simulink model "PIDcontroler"  (R2025b)
settings: Solver=VariableStepAuto  StartTime=0.0  StopTime=100  RelTol=1e-3
undefined symbols (not defined in the file): C_T_pitch, C_T_rol, C_T_yaw, Ix, Iy, Iz
libraries: slpidlib x3
settings Model: Creator=torcik  LastModifiedBy=torcik

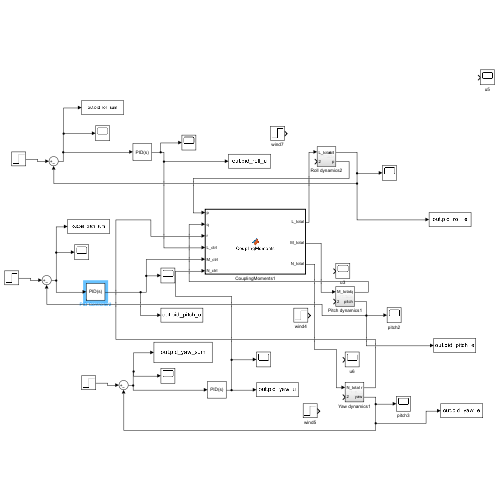
[thumbnail: Simulink's stored preview of the top-level diagram]
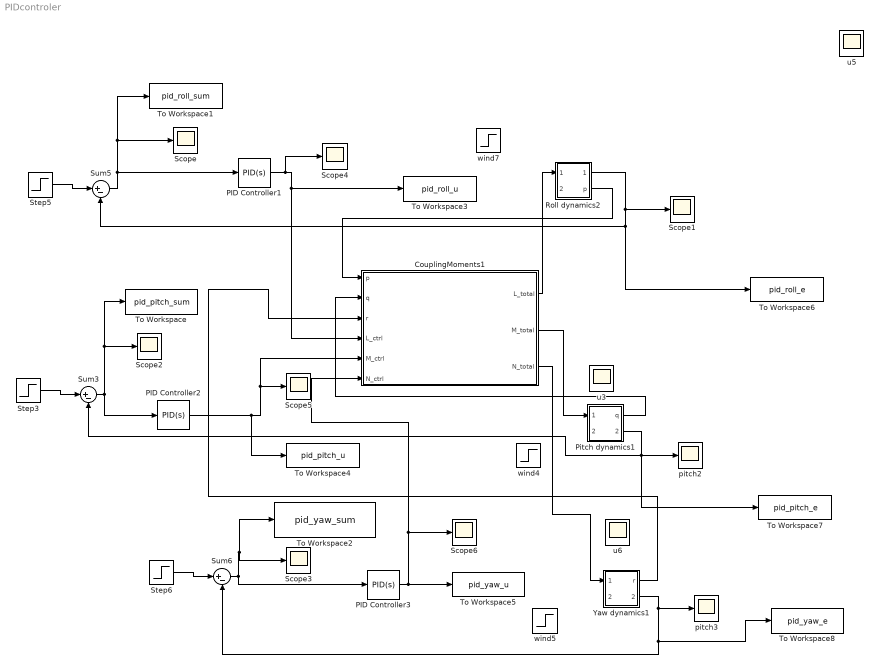
== system PIDcontroler ==
  CouplingMoments1 : MATLAB Function  TreatAsAtomicUnit=on
  PID Controller1 : slpidlib/PID Controller  Controller=PID  Form=Parallel  TimeDomain=Continuous-time  UseExternalTs=off  SampleTime=-1  IntegratorMethod=Forward Euler  FilterMethod=Forward Euler  ControllerParametersSource=internal  P=6.65  I=0.14  UseKiTs=off  D=15.6  UseExternalDerivativeSource=off  N=100  UseFilter=on  TunerSelectOption=Transfer Function Based (PID Tuner App)  InitialConditionSource=internal  InitialConditionForIntegrator=0  InitialConditionForFilter=0  DifferentiatorICPrevScaledInput=0  ExternalReset=none  TrackingMode=off  Kt=1  LimitOutput=off  SatLimitsSource=internal  UpperSaturationLimit=inf  LowerSaturationLimit=-inf  LinearizeAsGain=on  AntiWindupMode=none  Kb=1  LimitIntegrator=off  UpperIntegratorSaturationLimit=inf  LowerIntegratorSaturationLimit=-inf  POutMin=[]  POutMax=[]  IOutMin=[]  IOutMax=[]  DOutMin=[]  DOutMax=[]  NOutMin=[]  NOutMax=[]  SumOutMin=[]  SumOutMax=[]  SaturationOutMin=[]  SaturationOutMax=[]  PParamMin=[]  PParamMax=[]  IParamMin=[]  IParamMax=[]  DParamMin=[]  DParamMax=[]  NParamMin=[]  NParamMax=[]  KbParamMin=[]  KbParamMax=[]  KtParamMin=[]  KtParamMax=[]  KbOutMin=[]  KbOutMax=[]  KtOutMin=[]  KtOutMax=[]  IntegratorOutMin=[]  IntegratorOutMax=[]  FilterOutMin=[]  FilterOutMax=[]  SumI1OutMin=[]  SumI1OutMax=[]  SumI2OutMin=[]  SumI2OutMax=[]  SumI3OutMin=[]  SumI3OutMax=[]  SumI4OutMin=[]  SumI4OutMax=[]  SumDOutMin=[]  SumDOutMax=[]  DifferentiatorOutMin=[]  DifferentiatorOutMax=[]  FilterDiffOutCoefMin=[]  FilterDiffOutCoefMax=[]  ReciprocalOutMin=[]  ReciprocalOutMax=[]  SumDenOutMin=[]  SumDenOutMax=[]  SumNumOutMin=[]  SumNumOutMax=[]  DivideOutMin=[]  DivideOutMax=[]  UdiffTsProdOutMin=[]  UdiffTsProdOutMax=[]  NTsProdOutMin=[]  NTsProdOutMax=[]  UintegralTsProdOutMin=[]  UintegralTsProdOutMax=[]  UngainTsProdOutMin=[]  UngainTsProdOutMax=[]  ClampingZeroOutDataTypeStr=Inherit: Inherit via back propagation  ClampingZeroOutMin=[]  ClampingZeroOutMax=[]  FilterDenConstantOutDataTypeStr=Inherit: Inherit via back propagation  FilterDenConstantOutMin=[]  FilterDenConstantOutMax=[]  PCopyOutDataTypeStr=Inherit: Inherit via back propagation  PCopyOutMin=[]  PCopyOutMax=[]  NCopyOutDataTypeStr=Inherit: Inherit via back propagation  NCopyOutMin=[]  NCopyOutMax=[]  IntegratorContinuousStateAttributes=''  IntegratorStateMustResolveToSignalObject=off  IntegratorRTWStateStorageClass=Auto  FilterContinuousStateAttributes=''  FilterStateMustResolveToSignalObject=off  FilterRTWStateStorageClass=Auto  ParallelPVariant=InternalParameters  IdealPVariant=Disabled  IVariant=InternalParameters  DVariant=InternalParameters  IntegratorVariant=Continuous  SatVariant=Disabled  AWVariant=Passthrough  PCopyVariant=Disabled  TRVariant=Disabled  FdbkBlocksVariant=Forward  IdealPFdbkVariant=Disabled  SatFdbkVariant=Disabled  DerivativeFilterVariant=ContFilter  NVariant=InternalParameters  NCopyVariant=Disabled  FilterICVariant=InternalICsFilter  IntegratorICVariant=InternalICs  ExternalResetVariant=Disabled  TRSumVariant=Passthrough  SumFdbkVariant=Disabled  SumVariant=Sum_PID  TsampFilterVariant=InternalTs  TsampNgainVariant=Passthrough  TsampIntegralVariant=Disabled_SignalSpec  ExternalSaturationOutDataTypeStr=Inherit: Same as second input  DerivativeSourceVariant=ErrorSignal  PreIntVariant=InternalPreInt
  PID Controller2 : slpidlib/PID Controller  Controller=PID  Form=Parallel  TimeDomain=Continuous-time  UseExternalTs=off  SampleTime=-1  IntegratorMethod=Forward Euler  FilterMethod=Forward Euler  ControllerParametersSource=internal  P=9.74  I=0.17  UseKiTs=off  D=18.31  UseExternalDerivativeSource=off  N=100  UseFilter=on  TunerSelectOption=Transfer Function Based (PID Tuner App)  InitialConditionSource=internal  InitialConditionForIntegrator=0  InitialConditionForFilter=0  DifferentiatorICPrevScaledInput=0  ExternalReset=none  TrackingMode=off  Kt=1  LimitOutput=off  SatLimitsSource=internal  UpperSaturationLimit=inf  LowerSaturationLimit=-inf  LinearizeAsGain=on  AntiWindupMode=none  Kb=1  LimitIntegrator=off  UpperIntegratorSaturationLimit=inf  LowerIntegratorSaturationLimit=-inf  POutMin=[]  POutMax=[]  IOutMin=[]  IOutMax=[]  DOutMin=[]  DOutMax=[]  NOutMin=[]  NOutMax=[]  SumOutMin=[]  SumOutMax=[]  SaturationOutMin=[]  SaturationOutMax=[]  PParamMin=[]  PParamMax=[]  IParamMin=[]  IParamMax=[]  DParamMin=[]  DParamMax=[]  NParamMin=[]  NParamMax=[]  KbParamMin=[]  KbParamMax=[]  KtParamMin=[]  KtParamMax=[]  KbOutMin=[]  KbOutMax=[]  KtOutMin=[]  KtOutMax=[]  IntegratorOutMin=[]  IntegratorOutMax=[]  FilterOutMin=[]  FilterOutMax=[]  SumI1OutMin=[]  SumI1OutMax=[]  SumI2OutMin=[]  SumI2OutMax=[]  SumI3OutMin=[]  SumI3OutMax=[]  SumI4OutMin=[]  SumI4OutMax=[]  SumDOutMin=[]  SumDOutMax=[]  DifferentiatorOutMin=[]  DifferentiatorOutMax=[]  FilterDiffOutCoefMin=[]  FilterDiffOutCoefMax=[]  ReciprocalOutMin=[]  ReciprocalOutMax=[]  SumDenOutMin=[]  SumDenOutMax=[]  SumNumOutMin=[]  SumNumOutMax=[]  DivideOutMin=[]  DivideOutMax=[]  UdiffTsProdOutMin=[]  UdiffTsProdOutMax=[]  NTsProdOutMin=[]  NTsProdOutMax=[]  UintegralTsProdOutMin=[]  UintegralTsProdOutMax=[]  UngainTsProdOutMin=[]  UngainTsProdOutMax=[]  ClampingZeroOutDataTypeStr=Inherit: Inherit via back propagation  ClampingZeroOutMin=[]  ClampingZeroOutMax=[]  FilterDenConstantOutDataTypeStr=Inherit: Inherit via back propagation  FilterDenConstantOutMin=[]  FilterDenConstantOutMax=[]  PCopyOutDataTypeStr=Inherit: Inherit via back propagation  PCopyOutMin=[]  PCopyOutMax=[]  NCopyOutDataTypeStr=Inherit: Inherit via back propagation  NCopyOutMin=[]  NCopyOutMax=[]  IntegratorContinuousStateAttributes=''  IntegratorStateMustResolveToSignalObject=off  IntegratorRTWStateStorageClass=Auto  FilterContinuousStateAttributes=''  FilterStateMustResolveToSignalObject=off  FilterRTWStateStorageClass=Auto  ParallelPVariant=InternalParameters  IdealPVariant=Disabled  IVariant=InternalParameters  DVariant=InternalParameters  IntegratorVariant=Continuous  SatVariant=Disabled  AWVariant=Passthrough  PCopyVariant=Disabled  TRVariant=Disabled  FdbkBlocksVariant=Forward  IdealPFdbkVariant=Disabled  SatFdbkVariant=Disabled  DerivativeFilterVariant=ContFilter  NVariant=InternalParameters  NCopyVariant=Disabled  FilterICVariant=InternalICsFilter  IntegratorICVariant=InternalICs  ExternalResetVariant=Disabled  TRSumVariant=Passthrough  SumFdbkVariant=Disabled  SumVariant=Sum_PID  TsampFilterVariant=InternalTs  TsampNgainVariant=Passthrough  TsampIntegralVariant=Disabled_SignalSpec  ExternalSaturationOutDataTypeStr=Inherit: Same as second input  DerivativeSourceVariant=ErrorSignal  PreIntVariant=InternalPreInt
  PID Controller3 : slpidlib/PID Controller  Controller=PID  Form=Parallel  TimeDomain=Continuous-time  UseExternalTs=off  SampleTime=-1  IntegratorMethod=Forward Euler  FilterMethod=Forward Euler  ControllerParametersSource=internal  P=6.65  I=0.11  UseKiTs=off  D=18.75  UseExternalDerivativeSource=off  N=100  UseFilter=on  TunerSelectOption=Transfer Function Based (PID Tuner App)  InitialConditionSource=internal  InitialConditionForIntegrator=0  InitialConditionForFilter=0  DifferentiatorICPrevScaledInput=0  ExternalReset=none  TrackingMode=off  Kt=1  LimitOutput=off  SatLimitsSource=internal  UpperSaturationLimit=inf  LowerSaturationLimit=-inf  LinearizeAsGain=on  AntiWindupMode=none  Kb=1  LimitIntegrator=off  UpperIntegratorSaturationLimit=inf  LowerIntegratorSaturationLimit=-inf  POutMin=[]  POutMax=[]  IOutMin=[]  IOutMax=[]  DOutMin=[]  DOutMax=[]  NOutMin=[]  NOutMax=[]  SumOutMin=[]  SumOutMax=[]  SaturationOutMin=[]  SaturationOutMax=[]  PParamMin=[]  PParamMax=[]  IParamMin=[]  IParamMax=[]  DParamMin=[]  DParamMax=[]  NParamMin=[]  NParamMax=[]  KbParamMin=[]  KbParamMax=[]  KtParamMin=[]  KtParamMax=[]  KbOutMin=[]  KbOutMax=[]  KtOutMin=[]  KtOutMax=[]  IntegratorOutMin=[]  IntegratorOutMax=[]  FilterOutMin=[]  FilterOutMax=[]  SumI1OutMin=[]  SumI1OutMax=[]  SumI2OutMin=[]  SumI2OutMax=[]  SumI3OutMin=[]  SumI3OutMax=[]  SumI4OutMin=[]  SumI4OutMax=[]  SumDOutMin=[]  SumDOutMax=[]  DifferentiatorOutMin=[]  DifferentiatorOutMax=[]  FilterDiffOutCoefMin=[]  FilterDiffOutCoefMax=[]  ReciprocalOutMin=[]  ReciprocalOutMax=[]  SumDenOutMin=[]  SumDenOutMax=[]  SumNumOutMin=[]  SumNumOutMax=[]  DivideOutMin=[]  DivideOutMax=[]  UdiffTsProdOutMin=[]  UdiffTsProdOutMax=[]  NTsProdOutMin=[]  NTsProdOutMax=[]  UintegralTsProdOutMin=[]  UintegralTsProdOutMax=[]  UngainTsProdOutMin=[]  UngainTsProdOutMax=[]  ClampingZeroOutDataTypeStr=Inherit: Inherit via back propagation  ClampingZeroOutMin=[]  ClampingZeroOutMax=[]  FilterDenConstantOutDataTypeStr=Inherit: Inherit via back propagation  FilterDenConstantOutMin=[]  FilterDenConstantOutMax=[]  PCopyOutDataTypeStr=Inherit: Inherit via back propagation  PCopyOutMin=[]  PCopyOutMax=[]  NCopyOutDataTypeStr=Inherit: Inherit via back propagation  NCopyOutMin=[]  NCopyOutMax=[]  IntegratorContinuousStateAttributes=''  IntegratorStateMustResolveToSignalObject=off  IntegratorRTWStateStorageClass=Auto  FilterContinuousStateAttributes=''  FilterStateMustResolveToSignalObject=off  FilterRTWStateStorageClass=Auto  ParallelPVariant=InternalParameters  IdealPVariant=Disabled  IVariant=InternalParameters  DVariant=InternalParameters  IntegratorVariant=Continuous  SatVariant=Disabled  AWVariant=Passthrough  PCopyVariant=Disabled  TRVariant=Disabled  FdbkBlocksVariant=Forward  IdealPFdbkVariant=Disabled  SatFdbkVariant=Disabled  DerivativeFilterVariant=ContFilter  NVariant=InternalParameters  NCopyVariant=Disabled  FilterICVariant=InternalICsFilter  IntegratorICVariant=InternalICs  ExternalResetVariant=Disabled  TRSumVariant=Passthrough  SumFdbkVariant=Disabled  SumVariant=Sum_PID  TsampFilterVariant=InternalTs  TsampNgainVariant=Passthrough  TsampIntegralVariant=Disabled_SignalSpec  ExternalSaturationOutDataTypeStr=Inherit: Same as second input  DerivativeSourceVariant=ErrorSignal  PreIntVariant=InternalPreInt
  Pitch dynamics1 : Subsystem
  Roll dynamics2 : Subsystem
  Scope{,1..6} (7 alike) : Scope
      Scope settings: ActiveDisplayYMinimum=-31.219672370156161  ActiveDisplayYMaximum=28.315628159206881
      Scope1 settings: ActiveDisplayYMinimum=-37.930376847972084  ActiveDisplayYMaximum=31.772480353649549
      Scope2 settings: ActiveDisplayYMinimum=-41.5925552795621  ActiveDisplayYMaximum=35.188318402159311  DataLoggingVariableName=ScopeData3
      Scope3 settings: ActiveDisplayYMinimum=-49.309981749366955  ActiveDisplayYMaximum=52.967344378802764  DataLoggingVariableName=ScopeData2
      Scope4 settings: ActiveDisplayYMinimum=-197.56260181102388  ActiveDisplayYMaximum=186.16590351085537  DataLoggingVariableName=ScopeData4
      Scope5 settings: ActiveDisplayYMinimum=-3347.8386477727495  ActiveDisplayYMaximum=5841.9684075139066  DataLoggingVariableName=ScopeData5
      Scope6 settings: DataLoggingVariableName=ScopeData6
  Step3 : Step  After=10  SampleTime=0
  Step5 : Step  After=10  SampleTime=0
  Step6 : Step  After=10  SampleTime=0
  Sum3 : Sum  Inputs=|+-
  Sum5 : Sum  Inputs=|+-
  Sum6 : Sum  Inputs=|+-
  To Workspace : ToWorkspace  VariableName=pid_pitch_sum  SaveFormat=Timeseries  SampleTime=-1
  To Workspace1 : ToWorkspace  VariableName=pid_roll_sum  SaveFormat=Timeseries  SampleTime=-1
  To Workspace2 : ToWorkspace  VariableName=pid_yaw_sum  SaveFormat=Timeseries  SampleTime=-1
  To Workspace3 : ToWorkspace  VariableName=pid_roll_u  SaveFormat=Timeseries  SampleTime=-1
  To Workspace4 : ToWorkspace  VariableName=pid_pitch_u  SaveFormat=Timeseries  SampleTime=-1
  To Workspace5 : ToWorkspace  VariableName=pid_yaw_u  SaveFormat=Timeseries  SampleTime=-1
  To Workspace6 : ToWorkspace  VariableName=pid_roll_e  SaveFormat=Timeseries  SampleTime=-1
  To Workspace7 : ToWorkspace  VariableName=pid_pitch_e  SaveFormat=Timeseries  SampleTime=-1
  To Workspace8 : ToWorkspace  VariableName=pid_yaw_e  SaveFormat=Timeseries  SampleTime=-1
  Yaw dynamics1 : Subsystem
  pitch2 : Scope
      settings: ActiveDisplayYMinimum=-181.94758711954077  ActiveDisplayYMaximum=150.09620647460432  DataLoggingVariableName=ScopeData17
  pitch3 : Scope
      settings: ActiveDisplayYMinimum=-338.99297513586737  ActiveDisplayYMaximum=351.30222416565277  DataLoggingVariableName=ScopeData18
  u3 : Scope
      settings: ActiveDisplayYMinimum=-325.58366360782367  ActiveDisplayYMaximum=278.9525276257537  DataLoggingVariableName=ScopeData26
  u5 : Scope
      settings: ActiveDisplayYMinimum=-296.13255579071011  ActiveDisplayYMaximum=252.19959045289744  DataLoggingVariableName=ScopeData27
  u6 : Scope
      settings: ActiveDisplayYMinimum=-325.58366360782367  ActiveDisplayYMaximum=278.9525276257537  DataLoggingVariableName=ScopeData29
  wind4 : Step  Time=10  After=0  SampleTime=0
  wind5 : Step  Time=10  After=5  SampleTime=0
  wind7 : Step  Time=10  After=5  SampleTime=0
  wires:
  PID Controller3/1 -> Scope6/1, CouplingMoments1/6(N_ctrl), To Workspace5/1
  Pitch dynamics1/1(q) -> CouplingMoments1/2(q)
  Step3/1 -> Sum3/1
  Sum5/1 -> To Workspace1/1, Scope/1, PID Controller1/1
  CouplingMoments1/1(L_total) -> Roll dynamics2/1(L_total)
  CouplingMoments1/2(M_total) -> Pitch dynamics1/1(M_total)
  Roll dynamics2/2(p) -> CouplingMoments1/1(p)
  Roll dynamics2/1(roll) -> Scope1/1, To Workspace6/1, Sum5/2
  Step6/1 -> Sum6/1
  Yaw dynamics1/2(yaw) -> To Workspace8/1, Sum6/2, pitch3/1
  CouplingMoments1/3(N_total) -> Yaw dynamics1/1(N_total)
  Step5/1 -> Sum5/1
  Pitch dynamics1/2(pitch) -> To Workspace7/1, Sum3/2, pitch2/1
  Yaw dynamics1/1(r) -> CouplingMoments1/3(r)
  Sum6/1 -> To Workspace2/1, Scope3/1, PID Controller3/1
  Sum3/1 -> PID Controller2/1, Scope2/1, To Workspace/1
  PID Controller2/1 -> To Workspace4/1, CouplingMoments1/5(M_ctrl), Scope5/1
  PID Controller1/1 -> Scope4/1, CouplingMoments1/4(L_ctrl), To Workspace3/1

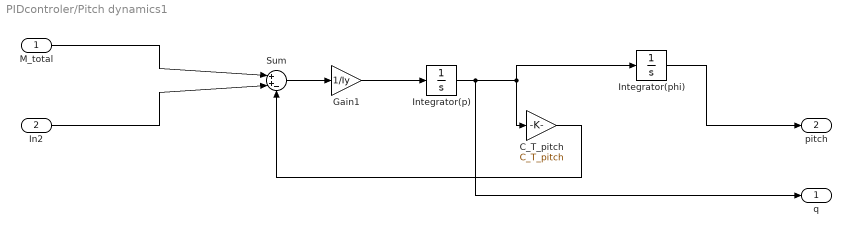
== system PIDcontroler/Pitch dynamics1 ==
  M_total : Inport
  In2 : Inport  Port=2
  C_T_pitch : Gain  Gain=C_T_pitch
  Gain1 : Gain  Gain=1/Iy
  Integrator(p) : Integrator
  Integrator(phi) : Integrator
  Sum : Sum  Inputs=|++-
  q : Outport
  pitch : Outport  Port=2
  wires:
  Integrator(p)/1 -> q/1, Integrator(phi)/1, C_T_pitch/1
  C_T_pitch/1 -> Sum/3
  Integrator(phi)/1 -> pitch/1
  Gain1/1 -> Integrator(p)/1
  M_total/1 -> Sum/1
  Sum/1 -> Gain1/1
  In2/1 -> Sum/2

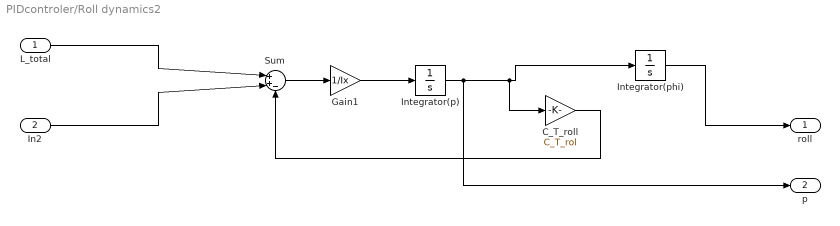
== system PIDcontroler/Roll dynamics2 ==
  L_total : Inport
  In2 : Inport  Port=2
  C_T_roll : Gain  Gain=C_T_rol
  Gain1 : Gain  Gain=1/Ix
  Integrator(p) : Integrator
  Integrator(phi) : Integrator
  Sum : Sum  Inputs=|++-
  roll : Outport
  p : Outport  Port=2
  wires:
  Integrator(p)/1 -> p/1, Integrator(phi)/1, C_T_roll/1
  C_T_roll/1 -> Sum/3
  Integrator(phi)/1 -> roll/1
  Gain1/1 -> Integrator(p)/1
  L_total/1 -> Sum/1
  Sum/1 -> Gain1/1
  In2/1 -> Sum/2

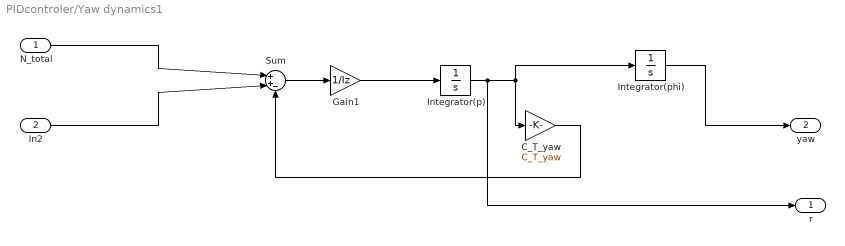
== system PIDcontroler/Yaw dynamics1 ==
  N_total : Inport
  In2 : Inport  Port=2
  C_T_yaw : Gain  Gain=C_T_yaw
  Gain1 : Gain  Gain=1/Iz
  Integrator(p) : Integrator
  Integrator(phi) : Integrator
  Sum : Sum  Inputs=|++-
  r : Outport
  yaw : Outport  Port=2
  wires:
  Integrator(p)/1 -> r/1, Integrator(phi)/1, C_T_yaw/1
  C_T_yaw/1 -> Sum/3
  Integrator(phi)/1 -> yaw/1
  Gain1/1 -> Integrator(p)/1
  N_total/1 -> Sum/1
  Sum/1 -> Gain1/1
  In2/1 -> Sum/2

== matlab function PIDcontroler/CouplingMoments1 ==
  data: p input; L_total output; q input; r input; L_ctrl input; M_ctrl input; N_ctrl input; M_total output; N_total output
function [L_total, M_total, N_total] = CouplingMoments(p, q, r, L_ctrl, M_ctrl, N_ctrl)


Ix = 100;     
Iy = 150;     
Iz = 200;  


L_coup = (Iy - Iz) * q * r;
M_coup = (Iz - Ix) * p * r;
N_coup = (Ix - Iy) * p * q;



L_total = L_ctrl + L_coup;
M_total = M_ctrl + M_coup;
N_total = N_ctrl + N_coup;
end
